simulink model "observer"  (R2021a)
settings: Solver=VariableStepAuto  StartTime=0.0  StopTime=2  RelTol=1e-3
values from neighbouring files (symbols this model uses):
  A = [0 0 0 0 0 1 -0.0174048595758 0 -0.0173759205618 -232.025201375 0 20.7861247087 ... (25 elements, 5x5)]    [matlab.mat]
  A_obs = A - B*K - L*C    [lab1_observer.m]    (also in varia_ganhos.m)
  B = [0 0 0 0 333.33674813]    [matlab.mat]
  B_obs = L    [lab1_observer.m]    (also in varia_ganhos.m)
  C = diag([1,1,1,1,1])    [lab1_observer.m]    (also in matlab.mat = [1 0 0 0 0 0 1 0 0 0 0 0 ... (25 elements, 5x5)]; varia_ganhos.m = eye(5))
  C_obs = -K    [lab1_observer.m]    (also in varia_ganhos.m)
  D = zeros(1)    [lab1.m]    (also in lab1_observer.m = [0 0 0 0 0]'; matlab.mat = [0 0 0 0 0]; varia_ganhos.m = [0 0 0 0 0]')
  D_obs = [0 0 0 0 0]    [lab1_observer.m]    (also in varia_ganhos.m = [0 0])
  x0 = [0.1 0 0 0 0]'    [lab1_observer.m]    (also in lab1_sim.m; matlab.mat = [0.1 0 0 0 0]; varia_ganhos.m)
settings Model: Creator=André  LastModifiedBy=André
settings DataIOCC: SaveOutput=off  SaveTime=off  ReturnWorkspaceOutputs=off

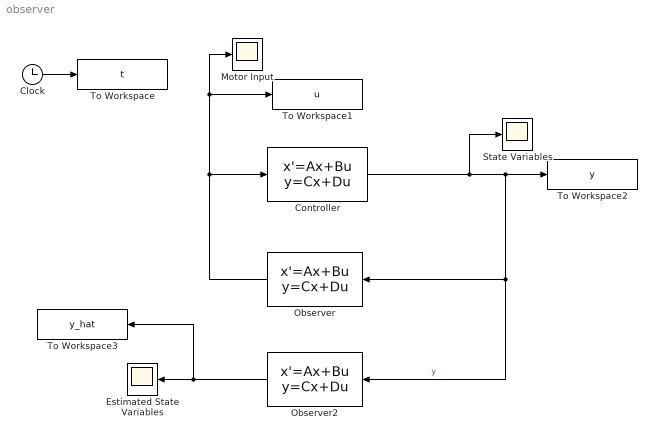
== system observer ==
  Clock : Clock
  Controller : StateSpace  A=A  B=B  C=C  D=D  InitialCondition=x0
  Estimated State Variables : Scope
  Motor Input : Scope
  Observer : StateSpace  A=A_obs  B=B_obs  C=C_obs  D=D_obs  InitialCondition=0
  Observer2 : StateSpace  A=A_obs  B=B_obs  C=diag([1,1,1,1,1])  D=diag([0,0,0,0,0])  InitialCondition=0
  State Variables : Scope
  To Workspace : ToWorkspace  VariableName=t  SampleTime=-1
  To Workspace1 : ToWorkspace  VariableName=u  SampleTime=-1
  To Workspace2 : ToWorkspace  VariableName=y  SampleTime=-1
  To Workspace3 : ToWorkspace  VariableName=y_hat  SampleTime=-1
  wires:
  Clock/1 -> To Workspace/1
  Controller/1 -> State Variables/1, To Workspace2/1, Observer2/1, Observer/1  "y"
  Observer/1 -> Motor Input/1, To Workspace1/1, Controller/1
  Observer2/1 -> To Workspace3/1, Estimated State Variables/1
